simulink model "Simulink_Electronico3"  (R2024a)
settings: Solver=VariableStepAuto  StartTime=0.0  StopTime=10.0  RelTol=1e-3
values from neighbouring files (symbols this model uses):
  C1 = 100e-6    (= 0.0001)    [Ec6.m]    (also in Simulink_Datos.m)
  C2 = 100e-6    (= 0.0001)    [Ec6.m]    (also in Simulink_Datos.m)
  R1 = 5e6    (= 5000000)    [Ec6.m]    (also in Simulink_Datos.m)
  R2 = 5e6    (= 5000000)    [Ec6.m]    (also in Simulink_Datos.m)
  R3 = 5e6    (= 5000000)    [Ec6.m]    (also in Simulink_Datos.m)
settings Model: Creator=Braulio Ramíreza  LastModifiedBy=Braulio Ramíreza

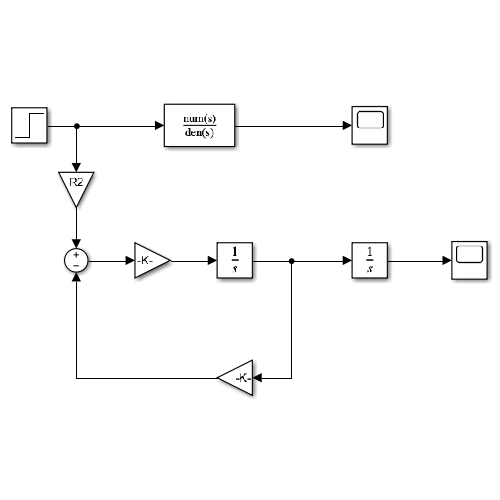
[thumbnail: Simulink's stored preview of the top-level diagram]
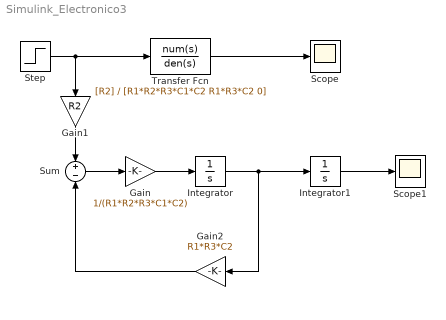
== system Simulink_Electronico3 ==
  Gain : Gain  Gain=1/(R1*R2*R3*C1*C2)
  Gain1 : Gain  Gain=R2
  Gain2 : Gain  Gain=R1*R3*C2
  Integrator : Integrator
  Integrator1 : Integrator
  Scope : Scope
  Scope1 : Scope
  Step : Step  Time=0  After=12  SampleTime=0
  Sum : Sum  Inputs=+-
  Transfer Fcn : TransferFcn  Numerator=[R2]  Denominator=[R1*R2*R3*C1*C2 R1*R3*C2 0]
  wires:
  Step/1 -> Gain1/1, Transfer Fcn/1
  Transfer Fcn/1 -> Scope/1
  Integrator/1 -> Gain2/1, Integrator1/1
  Gain/1 -> Integrator/1
  Sum/1 -> Gain/1
  Gain1/1 -> Sum/1
  Gain2/1 -> Sum/2
  Integrator1/1 -> Scope1/1
